simulink model "traffic_light"  (R2012b)
settings: Solver=ode45  StartTime=0.0  StopTime=10.0  RelTol=1e-3
settings Model: Creator=roberto  LastModifiedBy=roberto

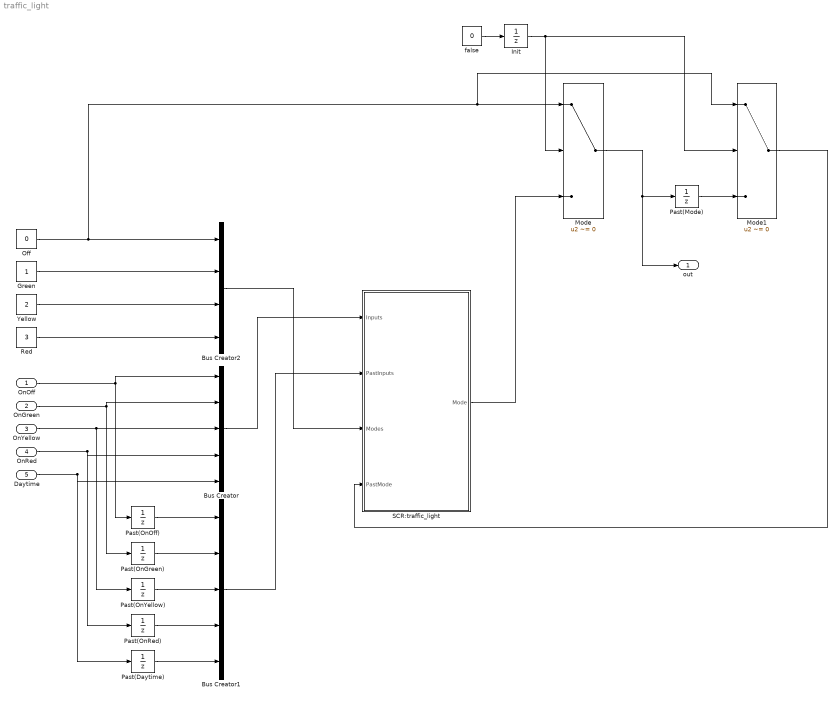
== system traffic_light ==
  OnOff : Inport  OutDataTypeStr=boolean
  OnGreen : Inport  Port=2  OutDataTypeStr=boolean
  OnYellow : Inport  Port=3  OutDataTypeStr=boolean
  OnRed : Inport  Port=4  OutDataTypeStr=boolean
  Daytime : Inport  Port=5  OutDataTypeStr=boolean
  Bus Creator : BusCreator  Inputs=5
  Bus Creator1 : BusCreator  Inputs=5
  Bus Creator2 : BusCreator
  Green : Constant  OutDataTypeStr=int8
  Init : UnitDelay  InitialCondition=1  SampleTime=-1
  Mode : Switch  Criteria=u2 ~= 0
  Mode1 : Switch  Criteria=u2 ~= 0
  Off : Constant  Value=0  OutDataTypeStr=int8
  Past(Daytime) : UnitDelay  InitialCondition=1  SampleTime=-1
  Past(Mode) : UnitDelay  InitialCondition=1  SampleTime=-1
  Past(OnGreen) : UnitDelay  InitialCondition=1  SampleTime=-1
  Past(OnOff) : UnitDelay  InitialCondition=1  SampleTime=-1
  Past(OnRed) : UnitDelay  InitialCondition=1  SampleTime=-1
  Past(OnYellow) : UnitDelay  InitialCondition=1  SampleTime=-1
  Red : Constant  Value=3  OutDataTypeStr=int8
  SCR:traffic_light : Subsystem
  Yellow : Constant  Value=2  OutDataTypeStr=int8
  false : Constant  Value=0  OutDataTypeStr=boolean
  out : Outport
  wires:
  false/1 -> Init/1
  Init/1 -> Mode1/2, Mode/2
  Off/1 -> Bus Creator2/1, Mode1/1, Mode/1
  OnOff/1 -> Past(OnOff)/1, Bus Creator/1
  OnGreen/1 -> Past(OnGreen)/1, Bus Creator/2
  OnYellow/1 -> Past(OnYellow)/1, Bus Creator/3
  OnRed/1 -> Past(OnRed)/1, Bus Creator/4
  Past(OnOff)/1 -> Bus Creator1/1
  Past(OnGreen)/1 -> Bus Creator1/2
  Past(OnYellow)/1 -> Bus Creator1/3
  Past(OnRed)/1 -> Bus Creator1/4
  Green/1 -> Bus Creator2/2
  Yellow/1 -> Bus Creator2/3
  Red/1 -> Bus Creator2/4
  Mode/1 -> out/1, Past(Mode)/1
  SCR:traffic_light/1(Mode) -> Mode/3
  Mode1/1 -> SCR:traffic_light/4(PastMode)
  Daytime/1 -> Past(Daytime)/1, Bus Creator/5
  Past(Daytime)/1 -> Bus Creator1/5
  Bus Creator2/1 -> SCR:traffic_light/3(Modes)
  Bus Creator/1 -> SCR:traffic_light/1(Inputs)
  Bus Creator1/1 -> SCR:traffic_light/2(PastInputs)
  Past(Mode)/1 -> Mode1/3

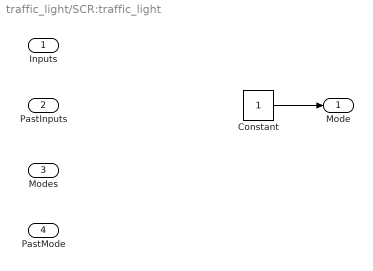
== system traffic_light/SCR:traffic_light ==
  Inputs : Inport
  PastInputs : Inport  Port=2
  Modes : Inport  Port=3
  PastMode : Inport  Port=4
  Constant : Constant  OutDataTypeStr=int8
  Mode : Outport
  wires:
  Constant/1 -> Mode/1
